simulink model "GradingSystem"  (R2021a)
settings: Solver=FixedStepDiscrete  StartTime=0.0  StopTime=10  RelTol=1e-3
settings Model: Creator=hp  LastModifiedBy=hp
settings OptimizationCC: DefaultParameterBehavior=Inlined  EnhancedBackFolding=on  PassReuseOutputArgsAs=Individual arguments  ZeroExternalMemoryAtStartup=off  ZeroInternalMemoryAtStartup=off  OptimizeBlockOrder=speed  DifferentSizesBufferReuse=on  OptimizationCustomize=off  EfficientTunableParamExpr=on
settings DebuggingCC: ParameterTunabilityLossMsg=error
settings SFSimCC: MATLABDynamicMemAlloc=off
settings RTWCC: SystemTargetFile=ert.tlc  GenCodeOnly=on  TemplateMakefile=ert_default_tmf  GenerateReport=on  IncludeHyperlinkInReport=on  LaunchReport=on  GenerateTraceInfo=on
settings CodeAppCC: ForceParamTrailComments=on  IgnoreCustomStorageClasses=off  OperatorAnnotations=on  SimulinkDataObjDesc=on  SFDataObjDesc=on  InsertBlockDesc=on
settings ERTTargetCC: TargetLangStandard=C99 (ISO)  GenerateSampleERTMain=on  SupportNonFinite=off  SupportComplex=off  InlinedParameterPlacement=NonHierarchical  ERTCustomFileTemplate=example_file_process.tlc  IndentSize=4  EnableUserReplacementTypes=on

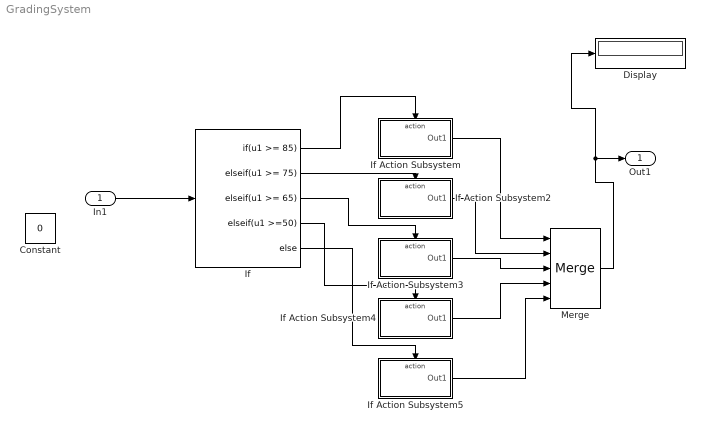
== system GradingSystem ==
  In1 : Inport  OutDataTypeStr=uint8
  Constant : Constant  Value=0
  Display : Display
  If : If  IfExpression=u1 >= 85  ElseIfExpressions=u1 >= 75, u1 >= 65, u1 >=50
  If Action Subsystem : Subsystem  TreatAsAtomicUnit=on
  If Action Subsystem2 : Subsystem  TreatAsAtomicUnit=on
  If Action Subsystem3 : Subsystem  TreatAsAtomicUnit=on
  If Action Subsystem4 : Subsystem  TreatAsAtomicUnit=on
  If Action Subsystem5 : Subsystem  TreatAsAtomicUnit=on
  Merge : Merge  Inputs=5
  Out1 : Outport
  wires:
  If Action Subsystem/1(Out1) -> Merge/1
  Merge/1 -> Display/1, Out1/1
  If/2 -> If Action Subsystem2/Action
  If/3 -> If Action Subsystem3/Action
  If/4 -> If Action Subsystem4/Action
  If/5 -> If Action Subsystem5/Action
  If/1 -> If Action Subsystem/Action
  If Action Subsystem2/1(Out1) -> Merge/2
  If Action Subsystem3/1(Out1) -> Merge/3
  If Action Subsystem4/1(Out1) -> Merge/4
  If Action Subsystem5/1(Out1) -> Merge/5
  In1/1 -> If/1

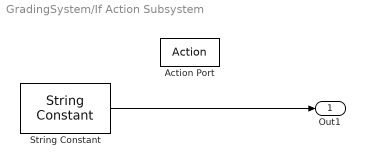
== system GradingSystem/If Action Subsystem ==
  Action Port : ActionPort  ActionPortLabel=if(u1 >= 85)
  String Constant : StringConstant  String="\"Excellent\""
  Out1 : Outport
  wires:
  String Constant/1 -> Out1/1

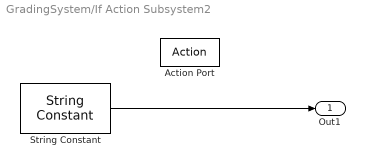
== system GradingSystem/If Action Subsystem2 ==
  Action Port : ActionPort  ActionPortLabel=elseif(u1 >= 75)
  String Constant : StringConstant  String="\"Very Good\""
  Out1 : Outport
  wires:
  String Constant/1 -> Out1/1

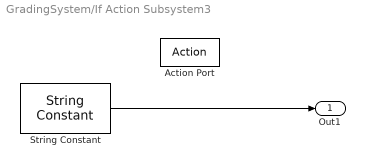
== system GradingSystem/If Action Subsystem3 ==
  Action Port : ActionPort  ActionPortLabel=elseif( u1 >= 65)
  String Constant : StringConstant  String="\"Good\""
  Out1 : Outport
  wires:
  String Constant/1 -> Out1/1

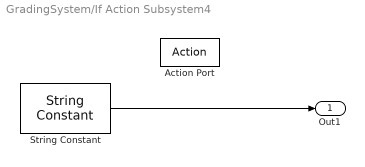
== system GradingSystem/If Action Subsystem4 ==
  Action Port : ActionPort  ActionPortLabel=elseif( u1 >=50)
  String Constant : StringConstant  String="\"Pass\""
  Out1 : Outport
  wires:
  String Constant/1 -> Out1/1

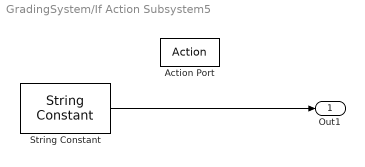
== system GradingSystem/If Action Subsystem5 ==
  Action Port : ActionPort  ActionPortLabel=else
  String Constant : StringConstant  String="\"Fail\""
  Out1 : Outport
  wires:
  String Constant/1 -> Out1/1
